simulink model "powerModule"  (R2018b)
settings: Solver=VariableStepAuto  StartTime=0.0  StopTime=10.0  RelTol=1e-3
undefined symbols (not defined in the file): Cdc, LdM, Lout, Rd, RdM
libraries: powerlib x17
settings Model: Creator=K2  LastModifiedBy=K2

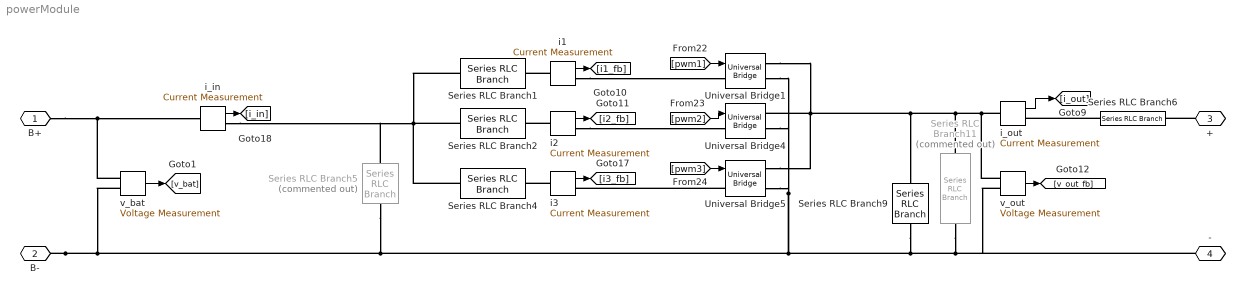
== system powerModule ==
  Series RLC Branch1 : powerlib/Elements/Series RLC Branch  LConnTagsString=__new0  RConnTagsString=__new0  BranchType=RL  Resistance=RdM(1)  Inductance=LdM(1)  SetiL0=off  InitialCurrent=0  Capacitance=100e-6  Setx0=off  InitialVoltage=0  Measurements=None
  Series RLC Branch11 : powerlib/Elements/Series RLC Branch  Commented=on  LConnTagsString=__new0  RConnTagsString=__new0  BranchType=Open circuit  Resistance=2000  Inductance=50e-6  SetiL0=off  InitialCurrent=0  Capacitance=100e-6  Setx0=off  InitialVoltage=0  Measurements=None
  Series RLC Branch2 : powerlib/Elements/Series RLC Branch  LConnTagsString=__new0  RConnTagsString=__new0  BranchType=RL  Resistance=RdM(2)  Inductance=LdM(2)  SetiL0=off  InitialCurrent=0  Capacitance=100e-6  Setx0=off  InitialVoltage=0  Measurements=None
  Series RLC Branch4 : powerlib/Elements/Series RLC Branch  LConnTagsString=__new0  RConnTagsString=__new0  BranchType=RL  Resistance=RdM(3)  Inductance=LdM(3)  SetiL0=off  InitialCurrent=0  Capacitance=100e-6  Setx0=off  InitialVoltage=0  Measurements=None
  Series RLC Branch5 : powerlib/Elements/Series RLC Branch  Commented=on  LConnTagsString=__new0  RConnTagsString=__new0  BranchType=C  Resistance=0.0001  Inductance=50e-6  SetiL0=off  InitialCurrent=0  Capacitance=8000e-6  Setx0=on  InitialVoltage=340  Measurements=None
  Series RLC Branch6 : powerlib/Elements/Series RLC Branch  LConnTagsString=__new0  RConnTagsString=__new0  BranchType=RL  Resistance=Rd  Inductance=Lout  SetiL0=off  InitialCurrent=0  Capacitance=1e-6  Setx0=off  InitialVoltage=0  Measurements=None
  Series RLC Branch9 : powerlib/Elements/Series RLC Branch  LConnTagsString=__new0  RConnTagsString=__new0  BranchType=C  Resistance=0.0001  Inductance=50e-6  SetiL0=off  InitialCurrent=0  Capacitance=Cdc  Setx0=on  InitialVoltage=550  Measurements=None
  Universal Bridge1 : powerlib/Power Electronics/Universal Bridge  Arms=1  SnubberResistance=1e5  SnubberCapacitance=inf  Device=MOSFET / Diodes  Ron=1e-3  Lon=0  ForwardVoltages="[  2  2  ]"  ForwardVoltage=0  GTOparameters=[ 10e-6 , 20e-6 ]  IGBTparameters=[ 1e-6 , 2e-6 ]  Measurements=None  Measurements_2=None  converterType=Rectifier
  Universal Bridge4 : powerlib/Power Electronics/Universal Bridge  Arms=1  SnubberResistance=1e5  SnubberCapacitance=inf  Device=MOSFET / Diodes  Ron=1e-3  Lon=0  ForwardVoltages="[  2  2  ]"  ForwardVoltage=0  GTOparameters=[ 10e-6 , 20e-6 ]  IGBTparameters=[ 1e-6 , 2e-6 ]  Measurements=None  Measurements_2=None  converterType=Rectifier
  Universal Bridge5 : powerlib/Power Electronics/Universal Bridge  Arms=1  SnubberResistance=1e5  SnubberCapacitance=inf  Device=MOSFET / Diodes  Ron=1e-3  Lon=0  ForwardVoltages="[  2  2  ]"  ForwardVoltage=0  GTOparameters=[ 10e-6 , 20e-6 ]  IGBTparameters=[ 1e-6 , 2e-6 ]  Measurements=None  Measurements_2=None  converterType=Rectifier
  i1 : powerlib/Measurements/Current Measurement  PhasorSimulation=off  OutputType=Complex  PSBequivalent=0
  i2 : powerlib/Measurements/Current Measurement  PhasorSimulation=off  OutputType=Complex  PSBequivalent=0
  i3 : powerlib/Measurements/Current Measurement  PhasorSimulation=off  OutputType=Complex  PSBequivalent=0
  i_in : powerlib/Measurements/Current Measurement  PhasorSimulation=off  OutputType=Complex  PSBequivalent=0
  i_out : powerlib/Measurements/Current Measurement  PhasorSimulation=off  OutputType=Complex  PSBequivalent=0
  v_bat : powerlib/Measurements/Voltage Measurement  PhasorSimulation=off  OutputType=Complex  PSBequivalent=0
  v_out : powerlib/Measurements/Voltage Measurement  PhasorSimulation=off  OutputType=Complex  PSBequivalent=0
  B+ : PMIOPort  Side=Left
  B- : PMIOPort  Port=2  Side=Left
  + : PMIOPort  Port=3  Side=Right
  - : PMIOPort  Port=4  Side=Right
  wires:
  i3/1 -> [i3_fb]
  v_out/1 -> [v_out_fb]
  [pwm2] -> Universal Bridge4/1
  v_bat/1 -> [v_bat]
  [pwm1] -> Universal Bridge1/1
  i_out/1 -> [i_out]
  i_in/1 -> [i_in]
  i1/1 -> [i1_fb]
  [pwm3] -> Universal Bridge5/1
  i2/1 -> [i2_fb]
  connections:
  v_bat/LConn1 -- i_in/LConn1 -- B+/RConn1
  B-/RConn1 -- v_bat/LConn2 -- Series RLC Branch5/RConn1 -- Series RLC Branch9/RConn1 -- Series RLC Branch11/RConn1 -- v_out/LConn2 -- -/RConn1 -- Universal Bridge5/RConn2 -- Universal Bridge1/RConn2 -- Universal Bridge4/RConn2
  i_out/LConn1 -- v_out/LConn1 -- Series RLC Branch11/LConn1 -- Series RLC Branch9/LConn1 -- Universal Bridge5/RConn1 -- Universal Bridge1/RConn1 -- Universal Bridge4/RConn1
  Series RLC Branch1/LConn1 -- Series RLC Branch4/LConn1 -- Series RLC Branch2/LConn1 -- i_in/RConn1 -- Series RLC Branch5/LConn1
  i2/RConn1 -- Universal Bridge4/LConn1
  Universal Bridge5/LConn1 -- i3/RConn1
  +/RConn1 -- Series RLC Branch6/LConn1
  i3/LConn1 -- Series RLC Branch4/RConn1
  i1/LConn1 -- Series RLC Branch1/RConn1
  i2/LConn1 -- Series RLC Branch2/RConn1
  i1/RConn1 -- Universal Bridge1/LConn1
  Series RLC Branch6/RConn1 -- i_out/RConn1
